simulink model "PID"  (R2022a)
settings: Solver=ode15s  StartTime=0.0  StopTime=10  RelTol=1e-3
libraries: slpidlib x1
settings Model: Creator=Adrii  LastModifiedBy=Adrian

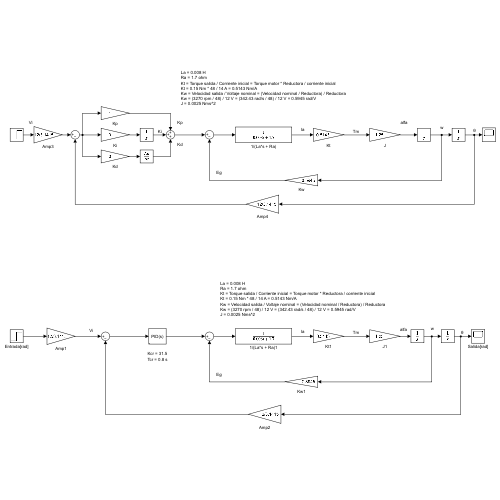
[thumbnail: Simulink's stored preview of the top-level diagram]
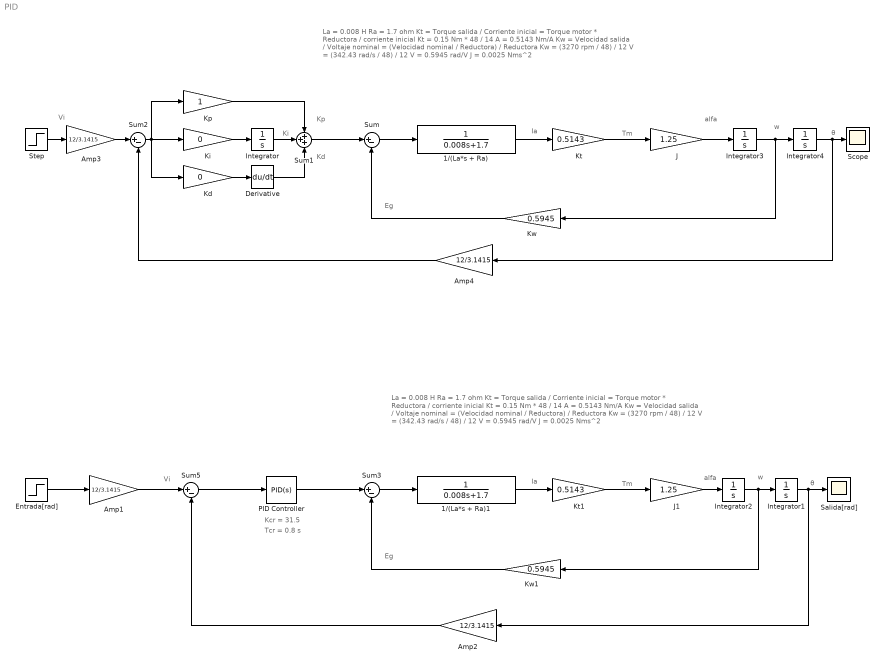
== system PID ==
  note: θ
  note: alfa
  note: Tcr = 0.8 s
  note: Kcr = 31.5
  note: alfa
  note: θ
  note: Kd
  note: Kp
  note: Ki
  note: w
  note: Vi
  note: Eg
  note: Tm
  note: Ia
  note: Tm
  note: Eg
  note: Ia
  note: La = 0.008 H
      | Ra = 1.7 ohm
      | Kt = Torque salida / Corriente inicial = Torque motor * Reductora / corriente inicial
      | Kt = 0.15 Nm * 48 / 14 A = 0.5143 Nm/A
      | Kw = Velocidad salida / Voltaje nominal = (Velocidad nominal / Reductora) / Reductora
      | Kw = (3270 rpm / 48) / 12 V = (342.43 rad/s / 48) / 12 V = 0.5945 rad/V
      | J = 0.0025 Nms^2
  note: Vi
  note: w
  note: La = 0.008 H
      | Ra = 1.7 ohm
      | Kt = Torque salida / Corriente inicial = Torque motor * Reductora / corriente inicial
      | Kt = 0.15 Nm * 48 / 14 A = 0.5143 Nm/A
      | Kw = Velocidad salida / Voltaje nominal = (Velocidad nominal / Reductora) / Reductora
      | Kw = (3270 rpm / 48) / 12 V = (342.43 rad/s / 48) / 12 V = 0.5945 rad/V
      | J = 0.0025 Nms^2
  1/(La*s + Ra) : TransferFcn  Denominator=[0.008 1.7]
  1/(La*s + Ra)1 : TransferFcn  Denominator=[0.008 1.7]
  Amp{1..4} (4 alike) : Gain  Gain=12/3.1415
  Derivative : Derivative
  Entrada[rad] : Step  Time=0  After=12  SampleTime=0
  Integrator{,1..4} (5 alike) : Integrator
  J : Gain  Gain=1.25
  J1 : Gain  Gain=1.25
  Kd : Gain  Gain=0
  Ki : Gain  Gain=0
  Kp : Gain
  Kt : Gain  Gain=0.5143
  Kt1 : Gain  Gain=0.5143
  Kw : Gain  Gain=0.5945
  Kw1 : Gain  Gain=0.5945
  PID Controller : slpidlib/PID Controller  Controller=PID  Form=Parallel  TimeDomain=Continuous-time  UseExternalTs=off  SampleTime=-1  IntegratorMethod=Forward Euler  FilterMethod=Forward Euler  ControllerParametersSource=internal  P=31.5  I=0  UseKiTs=off  D=0  N=100  UseFilter=on  TunerSelectOption=Transfer Function Based (PID Tuner App)  InitialConditionSource=internal  InitialConditionForIntegrator=0  InitialConditionForFilter=0  DifferentiatorICPrevScaledInput=0  ExternalReset=none  TrackingMode=off  Kt=1  LimitOutput=off  SatLimitsSource=internal  UpperSaturationLimit=inf  LowerSaturationLimit=-inf  LinearizeAsGain=on  AntiWindupMode=none  Kb=1  POutMin=[]  POutMax=[]  IOutMin=[]  IOutMax=[]  DOutMin=[]  DOutMax=[]  NOutMin=[]  NOutMax=[]  SumOutMin=[]  SumOutMax=[]  SaturationOutMin=[]  SaturationOutMax=[]  PParamMin=[]  PParamMax=[]  IParamMin=[]  IParamMax=[]  DParamMin=[]  DParamMax=[]  NParamMin=[]  NParamMax=[]  KbParamMin=[]  KbParamMax=[]  KtParamMin=[]  KtParamMax=[]  KbOutMin=[]  KbOutMax=[]  KtOutMin=[]  KtOutMax=[]  IntegratorOutMin=[]  IntegratorOutMax=[]  FilterOutMin=[]  FilterOutMax=[]  SumI1OutMin=[]  SumI1OutMax=[]  SumI2OutMin=[]  SumI2OutMax=[]  SumI3OutMin=[]  SumI3OutMax=[]  SumI4OutMin=[]  SumI4OutMax=[]  SumDOutMin=[]  SumDOutMax=[]  DifferentiatorOutMin=[]  DifferentiatorOutMax=[]  FilterDiffOutCoefMin=[]  FilterDiffOutCoefMax=[]  ReciprocalOutMin=[]  ReciprocalOutMax=[]  SumDenOutMin=[]  SumDenOutMax=[]  SumNumOutMin=[]  SumNumOutMax=[]  DivideOutMin=[]  DivideOutMax=[]  UdiffTsProdOutMin=[]  UdiffTsProdOutMax=[]  NTsProdOutMin=[]  NTsProdOutMax=[]  UintegralTsProdOutMin=[]  UintegralTsProdOutMax=[]  UngainTsProdOutMin=[]  UngainTsProdOutMax=[]  IntegratorContinuousStateAttributes=''  IntegratorStateMustResolveToSignalObject=off  IntegratorRTWStateStorageClass=Auto  FilterContinuousStateAttributes=''  FilterStateMustResolveToSignalObject=off  FilterRTWStateStorageClass=Auto  ParallelPVariant=InternalParameters  IdealPVariant=Disabled  IVariant=InternalParameters  DVariant=InternalParameters  IntegratorVariant=Continuous  SatVariant=Disabled  AWVariant=Passthrough  PCopyVariant=Disabled  TRVariant=Disabled  FdbkBlocksVariant=Forward  IdealPFdbkVariant=Disabled  SatFdbkVariant=Disabled  DerivativeFilterVariant=ContFilter  NVariant=InternalParameters  NCopyVariant=Disabled  FilterICVariant=InternalICsFilter  IntegratorICVariant=InternalICs  ExternalResetVariant=Disabled  TRSumVariant=Passthrough  SumFdbkVariant=Disabled  SumVariant=Sum_PID  TsampFilterVariant=InternalTs  TsampNgainVariant=Passthrough  TsampIntegralVariant=Passthrough  ExternalSaturationOutDataTypeStr=Inherit: Same as second input  aMode=0
  Salida[rad] : Scope
  Scope : Scope
  Step : Step  Time=0  SampleTime=0
  Sum{,2..3,5} (4 alike) : Sum  Inputs=|+-
  Sum1 : Sum  Inputs=+++
  wires:
  Kp/1 -> Sum1/1
  Kw/1 -> Sum/2
  1/(La*s + Ra)/1 -> Kt/1
  Kt/1 -> J/1
  Ki/1 -> Integrator/1
  Kd/1 -> Derivative/1
  Integrator/1 -> Sum1/2
  Derivative/1 -> Sum1/3
  Sum/1 -> 1/(La*s + Ra)/1
  Sum1/1 -> Sum/1
  Sum2/1 -> Kd/1, Kp/1, Ki/1
  Sum3/1 -> 1/(La*s + Ra)1/1
  Kt1/1 -> J1/1
  Kw1/1 -> Sum3/2
  1/(La*s + Ra)1/1 -> Kt1/1
  Sum5/1 -> PID Controller/1
  PID Controller/1 -> Sum3/1
  Integrator1/1 -> Amp2/1, Salida[rad]/1
  Amp2/1 -> Sum5/2
  Amp1/1 -> Sum5/1
  Entrada[rad]/1 -> Amp1/1
  J1/1 -> Integrator2/1
  Integrator2/1 -> Kw1/1, Integrator1/1
  Step/1 -> Amp3/1
  Amp3/1 -> Sum2/1
  J/1 -> Integrator3/1
  Integrator3/1 -> Kw/1, Integrator4/1
  Integrator4/1 -> Amp4/1, Scope/1
  Amp4/1 -> Sum2/2
